simulink model "PositionComplementary2"  (Simulink 6.6)
settings: Solver=ode4  StartTime=0.0  StopTime=1800  FixedStep=SampleT  RelTol=1e-3
InitFcn:
  | clc
  | Taxi_Var_new
  | failures
  | insInit
  | piccolo_init
values from neighbouring files (symbols this model uses):
  A1 = 0    [Taxi_Var.m]    (also in Taxi_Var_new.m = 0.007)
  Apolar = 0.0899    [Taxi_Var.m]    (also in Taxi_Var_new.m = 0.057)
  CD0 = 0.0219    [Taxi_Var.m]    (also in Taxi_Var_new.m = 0.022)
  chord = S/span    (= 0.384036716878)    [Taxi_Var.m]    (also in Taxi_Var_new.m = 0.351341681574)
  CL0 = 0.1857    [Taxi_Var.m]    (also in Taxi_Var_new.m = 0.38)
  CLa = 4.6206    [Taxi_Var.m]    (also in Taxi_Var_new.m = 18.5)
  CLa_dot = 1.93    [Taxi_Var.m]    (also in Taxi_Var_new.m = 2.64)
  Clb = -0.0043    [Taxi_Var.m]    (also in Taxi_Var_new.m = -0.06)
  ClDa = 0.1695    [Taxi_Var.m]    (also in Taxi_Var_new.m)
  CLDe = 0.4032    [Taxi_Var.m]    (also in Taxi_Var_new.m = 0.24)
  CLDf = 0.047    [Taxi_Var.m]    (also in Taxi_Var_new.m = 0.4)
  ClDr = 0.0003    [Taxi_Var.m]    (also in Taxi_Var_new.m = 0.055)
  Clp = -0.4425    [Taxi_Var.m]    (also in Taxi_Var_new.m = -0.88)
  CLq = 8.7465    [Taxi_Var.m]    (also in Taxi_Var_new.m = 7.4)
  Clr = 0.0675    [Taxi_Var.m]    (also in Taxi_Var_new.m = 0.04)
  Cm0 = -0.0902    [Taxi_Var.m]    (also in Taxi_Var_new.m = 0.56)
  Cma = -1.3995    [Taxi_Var.m]    (also in Taxi_Var_new.m = -1.58)
  CmDe = -0.9493    [Taxi_Var.m]    (also in Taxi_Var_new.m = -41)
  CmDf = -.021    (= -0.021)    [Taxi_Var.m]    (also in Taxi_Var_new.m)
  Cmq = -10.8760    (= -10.876)    [Taxi_Var.m]    (also in Taxi_Var_new.m = -12)
  Cnb = 0.0281    [Taxi_Var.m]    (also in Taxi_Var_new.m = 0.73)
  CnDa = -0.0031    [Taxi_Var.m]    (also in Taxi_Var_new.m = -0.032)
  CnDr = -0.0882    [Taxi_Var.m]    (also in Taxi_Var_new.m = 0.19)
  Cnp = -0.0695    [Taxi_Var.m]    (also in Taxi_Var_new.m = -0.1)
  Cnr = -0.1045    [Taxi_Var.m]    (also in Taxi_Var_new.m = -0.23)
  CYb = -0.1999    [Taxi_Var.m]    (also in Taxi_Var_new.m = -0.98)
  CYDr = 0.0192    [Taxi_Var.m]    (also in Taxi_Var_new.m = 0.066)
  damax = 25*deg2rad    (= 0.436332312999)    [Taxi_Var.m]    (also in piccolo_init.m)
  damin = -25*deg2rad    (= -0.436332312999)    [Taxi_Var.m]    (also in piccolo_init.m)
  datrim = 0*deg2rad    (= 0)    [Taxi_Var.m]    (also in piccolo_init.m)
  demax = 15*deg2rad    (= 0.261799387799)    [Taxi_Var.m]    (also in piccolo_init.m)
  demin = -15*deg2rad    (= -0.261799387799)    [Taxi_Var.m]    (also in piccolo_init.m)
  detrim = -2.4137*deg2rad    (= -0.0421270121554)    [Taxi_Var.m]    (also in piccolo_init.m = -0.0523598775598)
  dfland = 30*deg2rad    (= 0.523598775598)    [Taxi_Var.m]    (also in piccolo_init.m)
  dfmax = 30*deg2rad    (= 0.523598775598)    [Taxi_Var.m]    (also in piccolo_init.m)
  dfmin = 0*deg2rad    (= 0)    [Taxi_Var.m]    (also in piccolo_init.m)
  drmax = 25*deg2rad    (= 0.436332312999)    [Taxi_Var.m]    (also in piccolo_init.m)
  drmin = -25*deg2rad    (= -0.436332312999)    [Taxi_Var.m]    (also in piccolo_init.m)
  drtrim = 0*deg2rad    (= 0)    [Taxi_Var.m]    (also in piccolo_init.m)
  dtmax = 1    [Taxi_Var.m]    (also in piccolo_init.m = 0.7)
  dtmin = 0    [Taxi_Var.m]    (also in piccolo_init.m = 0.25)
  dttrim = 0.0725    [Taxi_Var.m]    (also in piccolo_init.m = 0.35)
  Euler_0 = [0; 0; 45]'*pi/180    [Taxi_Var.m]    (also in Taxi_Var_new.m = [0 0 45]'*pi/180)
  IdxCmdOrbitRadius = 17    [piccolo_init.m]
  IdxCmdOrbitSense = 18    [piccolo_init.m]
  IdxCmdWp1Alt = 13    [piccolo_init.m]
  IdxCmdWp1Lat = 11    [piccolo_init.m]
  IdxCmdWp1Lon = 12    [piccolo_init.m]
  IdxCmdWp2Alt = 16    [piccolo_init.m]
  IdxCmdWp2Lat = 14    [piccolo_init.m]
  IdxCmdWp2Lon = 15    [piccolo_init.m]
  IdxEstimReserved1 = 4    [piccolo_init.m]
  IdxEstimWEast = 3    [piccolo_init.m]
  IdxEstimWNorth = 2    [piccolo_init.m]
  IdxGainsAltD = 10    [piccolo_init.m]
  IdxGainsAltI = 9    [piccolo_init.m]
  IdxGainsAltP = 8    [piccolo_init.m]
  IdxGainsPdynD = 4    [piccolo_init.m]
  IdxGainsPdynI = 3    [piccolo_init.m]
  IdxGainsPdynP = 2    [piccolo_init.m]
  IdxGainsPitchD = 7    [piccolo_init.m]
  IdxGainsPitchI = 6    [piccolo_init.m]
  IdxGainsPitchP = 5    [piccolo_init.m]
  IdxGainsRollD = 17    [piccolo_init.m]
  IdxGainsRollI = 16    [piccolo_init.m]
  IdxGainsRollP = 15    [piccolo_init.m]
  IdxGainsSlopeElevatorD = 25    [piccolo_init.m]
  IdxGainsSlopeElevatorP = 26    [piccolo_init.m]
  IdxGainsTrackConv = 24    [piccolo_init.m]
  IdxGainsTrackD = 23    [piccolo_init.m]
  IdxGainsTrackI = 22    [piccolo_init.m]
  IdxGainsTrackP = 21    [piccolo_init.m]
  IdxGainsTurnD = 14    [piccolo_init.m]
  IdxGainsTurnI = 13    [piccolo_init.m]
  IdxGainsTurnP = 12    [piccolo_init.m]
  IdxGainsYawD = 20    [piccolo_init.m]
  IdxGainsYawI = 19    [piccolo_init.m]
  IdxGainsYawP = 18    [piccolo_init.m]
  IdxLimitsAileronMax = 11    [piccolo_init.m]
  IdxLimitsAileronMin = 10    [piccolo_init.m]
  IdxLimitsBankMax = 9    [piccolo_init.m]
  IdxLimitsBankMin = 8    [piccolo_init.m]
  IdxLimitsElevatorMax = 13    [piccolo_init.m]
  IdxLimitsElevatorMin = 12    [piccolo_init.m]
  IdxLimitsFlapMax = 19    [piccolo_init.m]
  IdxLimitsFlapMin = 18    [piccolo_init.m]
  IdxLimitsPdynMax = 3    [piccolo_init.m]
  IdxLimitsPdynMin = 2    [piccolo_init.m]
  IdxLimitsRudderMax = 15    [piccolo_init.m]
  IdxLimitsRudderMin = 14    [piccolo_init.m]
  IdxLimitsThrottleMax = 17    [piccolo_init.m]
  IdxLimitsThrottleMin = 16    [piccolo_init.m]
  IdxSensorsAlt = 5    [piccolo_init.m]
  IdxSensorsLat = 3    [piccolo_init.m]
  IdxSensorsLon = 4    [piccolo_init.m]
  IdxSensorsVDown = 8    [piccolo_init.m]
  IdxSensorsVEast = 7    [piccolo_init.m]
  IdxSensorsVNorth = 6    [piccolo_init.m]
  IdxStatesGlobal = 2    [piccolo_init.m]
  IdxStatesManual = 16    [piccolo_init.m]
  IdxStatesMode = 15    [piccolo_init.m]
  ISA_g = 9.815    [Taxi_Var.m]    (also in Taxi_Var_new.m)
  ISA_hmax = 2000    [Taxi_Var.m]    (also in Taxi_Var_new.m)
  ISA_lapse = .0065    (= 0.0065)    [Taxi_Var.m]    (also in Taxi_Var_new.m)
  ISA_P0 = 101325    [Taxi_Var.m]    (also in Taxi_Var_new.m)
  ISA_R = 287    [Taxi_Var.m]    (also in Taxi_Var_new.m)
  ISA_rho0 = 1.225    [Taxi_Var.m]    (also in Taxi_Var_new.m)
  ISA_T0 = 289    [Taxi_Var.m]    (also in Taxi_Var_new.m)
  Ixx = 3.689084    [Taxi_Var.m]    (also in Taxi_Var_new.m = 3.8)
  Iyy = 7.43789    [Taxi_Var.m]    (also in Taxi_Var_new.m = 9.58)
  Izz = 10.22202    [Taxi_Var.m]    (also in Taxi_Var_new.m = 9.68)
  mass = 22.5    [Taxi_Var.m]    (also in Taxi_Var_new.m = 8.16466266)
  MinThK = 0.075    [Taxi_Var.m]    (also in Taxi_Var_new.m = 0.077)
  Pos_0 = [0; 0; 1000]'    [Taxi_Var.m]    (also in Taxi_Var_new.m = [0 0 500]')
  PQR_0 = [0; 0; 0]'    [Taxi_Var.m]    (also in Taxi_Var_new.m = [ 0 0 0]'*pi/180)
  SampleT = 0.005    [failures.m]
  span = 2.3368    [Taxi_Var.m]    (also in Taxi_Var_new.m = 2.795)
  TFact = 0.4    [Taxi_Var.m]    (also in Taxi_Var_new.m)
  ThK = 2.18    [Taxi_Var.m]    (also in Taxi_Var_new.m = 2.17)
  tsamp = APtsamp    (= 0.05)    [piccolo_init.m]
  ... (+1 more)
undefined symbols (not defined in the file or in its folder): clock, DiscIntNeverNeededParam, Earth, gaind, polesd, WGS84, zerosd
libraries: piccolo_library x60, simulink x49, aerolibconvert2 x16, dspsigops x5, aerolibasang x5, aerolibatmos2 x2, aerolibtransform2 x2, aerolibnav x2, aerolibutil x1, dspmtrx3 x1
(part 2 of 6)

== system PositionComplementary2/Subsystem3/Autopilot ==
  Sensors : Inport  PortDimensions=SizeSensors
  Estimates : Inport  Port=2  PortDimensions=SizeEstim
  Settings : Inport  Port=3  PortDimensions=SizeSet
  Commands : Inport  Port=4  PortDimensions=SizeCmd
  States : Inport  Port=5  PortDimensions=SizeStates
  Gains : Inport  Port=6  PortDimensions=SizeGains
  Limits : Inport  Port=7  PortDimensions=SizeLimits
  Autopilot Enable : EnablePort  StatesWhenEnabling=reset
  Air System Vector Inputs : piccolo_library/Flight Mechanics/Air System Vector Inputs  SystemSampleTime=-1  tsamp=APtsamp
  Altitude Control Vector Inputs : Subsystem  AncestorBlock=piccolo_library/Controllers/Longitudinal/Altitude Control Vector Inputs
  Demux{,1..6} (7 alike) : Demux  Outputs=7
  Flap Control Vector Inputs : Subsystem
  Gain : Gain  SaturateOnIntegerOverflow=on
  Gain1 : Gain  SaturateOnIntegerOverflow=on
  Guidance & Navigation Vector Input : Subsystem  AncestorBlock=piccolo_library/Controllers/Guidance/Guidance & Navigation Vector Input
  Mux : Mux  Inputs=12
  Mux1 : Mux  Inputs=5
  Mux2 : Mux  Inputs=7
  Pitch Control  Vector Inputs : Subsystem  AncestorBlock="piccolo_library/Controllers/Longitudinal/Pitch Control  Vector Inputs"
  Reserved Outputs : Constant  Value=0
  Roll Control Vector Inputs : Subsystem  AncestorBlock=piccolo_library/Controllers/Lateral/Roll Control Vector Inputs
  Yaw Control Vector Inputs : Subsystem  AncestorBlock=piccolo_library/Controllers/Lateral/Yaw Control Vector Inputs
  Actuators : Outport  OutDataType=fixdt(1,16,0)  OutScaling=[]
  Derived : Outport  Port=2  OutDataType=fixdt(1,16,0)  OutScaling=[]
  NPSTrim : Outport  Port=3  OutDataType=fixdt(1,16,0)  OutScaling=[]  InitialOutput=0
  wires:
  Mux/1 -> Gain/1, NPSTrim/1
  Mux1/1 -> Roll Control Vector Inputs/8(Derived), Altitude Control Vector Inputs/8(Derived), Pitch Control  Vector Inputs/8(Derived), Guidance & Navigation Vector Input/8(Derived), Yaw Control Vector Inputs/8(Derived), Air System Vector Inputs/8, Flap Control Vector Inputs/8(Derived), Gain1/1
  Roll Control Vector Inputs/1(Actuator) -> Mux/2
  Pitch Control  Vector Inputs/1(Actuator) -> Mux/4
  Altitude Control Vector Inputs/1(Actuator) -> Mux/8
  Sensors/1 -> Mux2/1
  Estimates/1 -> Mux2/2
  Settings/1 -> Mux2/3
  Commands/1 -> Mux2/4
  States/1 -> Mux2/5
  Gains/1 -> Mux2/6
  Limits/1 -> Mux2/7
  Demux/1 -> Altitude Control Vector Inputs/1(Sensors)
  Demux/2 -> Altitude Control Vector Inputs/2(Estimates)
  Demux/3 -> Altitude Control Vector Inputs/3(Settings)
  Demux/4 -> Altitude Control Vector Inputs/4(Commands)
  Demux/5 -> Altitude Control Vector Inputs/5(States)
  Demux/6 -> Altitude Control Vector Inputs/6(Gains)
  Demux/7 -> Altitude Control Vector Inputs/7(Limits)
  Demux1/1 -> Roll Control Vector Inputs/1(Sensors)
  Demux1/2 -> Roll Control Vector Inputs/2(Estimates)
  Demux1/3 -> Roll Control Vector Inputs/3(Settings)
  Demux1/4 -> Roll Control Vector Inputs/4(Commands)
  Demux1/5 -> Roll Control Vector Inputs/5(States)
  Demux1/6 -> Roll Control Vector Inputs/6(Gains)
  Demux1/7 -> Roll Control Vector Inputs/7(Limits)
  Demux2/1 -> Pitch Control  Vector Inputs/1(Sensors)
  Demux2/2 -> Pitch Control  Vector Inputs/2(Estimates)
  Demux2/3 -> Pitch Control  Vector Inputs/3(Settings)
  Demux2/4 -> Pitch Control  Vector Inputs/4(Commands)
  Demux2/5 -> Pitch Control  Vector Inputs/5(States)
  Demux2/6 -> Pitch Control  Vector Inputs/6(Gains)
  Demux2/7 -> Pitch Control  Vector Inputs/7(Limits)
  Demux3/1 -> Guidance & Navigation Vector Input/1(Sensors)
  Demux3/2 -> Guidance & Navigation Vector Input/2(Estimates)
  Demux3/3 -> Guidance & Navigation Vector Input/3(Settings)
  Demux3/4 -> Guidance & Navigation Vector Input/4(Commands)
  Demux3/5 -> Guidance & Navigation Vector Input/5(States)
  Demux3/6 -> Guidance & Navigation Vector Input/6(Gains)
  Demux3/7 -> Guidance & Navigation Vector Input/7(Limits)
  Demux4/1 -> Yaw Control Vector Inputs/1(Sensors)
  Demux4/2 -> Yaw Control Vector Inputs/2(Estimates)
  Demux4/3 -> Yaw Control Vector Inputs/3(Settings)
  Demux4/4 -> Yaw Control Vector Inputs/4(Commands)
  Demux4/5 -> Yaw Control Vector Inputs/5(States)
  Demux4/6 -> Yaw Control Vector Inputs/6(Gains)
  Demux4/7 -> Yaw Control Vector Inputs/7(Limits)
  Demux5/1 -> Air System Vector Inputs/1
  Demux5/2 -> Air System Vector Inputs/2
  Demux5/3 -> Air System Vector Inputs/3
  Demux5/4 -> Air System Vector Inputs/4
  Demux5/5 -> Air System Vector Inputs/5
  Demux5/6 -> Air System Vector Inputs/6
  Demux5/7 -> Air System Vector Inputs/7
  Mux2/1 -> Demux1/1, Demux/1, Demux2/1, Demux3/1, Demux4/1, Demux5/1, Demux6/1
  Reserved Outputs/1 -> Mux/11, Mux/9, Mux/7, Mux/1, Mux/3, Mux/5, Mux/12
  Yaw Control Vector Inputs/1(Actuator) -> Mux/6
  Flap Control Vector Inputs/1(Actuator) -> Mux/10
  Demux6/1 -> Flap Control Vector Inputs/1(Sensors)
  Demux6/2 -> Flap Control Vector Inputs/2(Estimates)
  Demux6/3 -> Flap Control Vector Inputs/3(Settings)
  Demux6/4 -> Flap Control Vector Inputs/4(Commands)
  Demux6/5 -> Flap Control Vector Inputs/5(States)
  Demux6/6 -> Flap Control Vector Inputs/6(Gains)
  Demux6/7 -> Flap Control Vector Inputs/7(Limits)
  Air System Vector Inputs/1 -> Mux1/1
  Roll Control Vector Inputs/2(Param) -> Mux1/2
  Pitch Control  Vector Inputs/2(Param) -> Mux1/3
  Guidance & Navigation Vector Input/1(Param) -> Mux1/4
  Altitude Control Vector Inputs/2(Param) -> Mux1/5
  Gain/1 -> Actuators/1
  Gain1/1 -> Derived/1

== system PositionComplementary2/Subsystem3/L1 Adaptive Controller LATERAL-DIRECTIONAL ==
  u_psi_c : Inport
  u_psi : Inport  Port=2
  Display : Display
  Mux2 : Mux  Inputs=2
  PF Yaw Channel L1 Augmentation : Subsystem  Orientation=left
  Scope1 : Scope  NumInputPorts=2
      settings: YMin=0.0999875~-4.5e-005  YMax=0.100045~1.25e-005  SaveName=ScopeData28
  Sum1 : Sum  Inputs=-+|
  Sum2 : Sum  Inputs=-+|
  u2 : Outport
  wires:
  u_psi/1 -> PF Yaw Channel L1 Augmentation/1(u_psi), Mux2/2, Sum2/1
  PF Yaw Channel L1 Augmentation/1(C_sighat_2) -> Sum1/1, Display/1  "L1 augmentation"
  u_psi_c/1 -> Sum1/2, Mux2/1, Sum2/2
  Sum1/1 -> u2/1, PF Yaw Channel L1 Augmentation/2(u2)
  Mux2/1 -> Scope1/1
  Sum2/1 -> Scope1/2

== system PositionComplementary2/Subsystem3/L1 Adaptive Controller LONGITUDINAL ==
  u_psi_c : Inport
  u_psi : Inport  Port=2
  Display : Display
  Mux2 : Mux  Inputs=2
  PF Yaw Channel L1 Augmentation : Subsystem  Orientation=left
  Scope1 : Scope  NumInputPorts=2
      settings: YMin=0.0999875~-4.5e-005  YMax=0.100045~1.25e-005  SaveName=ScopeData28
  Sum1 : Sum  Inputs=-+|
  Sum2 : Sum  Inputs=-+|
  u2 : Outport
  wires:
  Sum2/1 -> Scope1/2
  Mux2/1 -> Scope1/1
  Sum1/1 -> PF Yaw Channel L1 Augmentation/2(u2), u2/1
  u_psi_c/1 -> Sum2/2, Mux2/1, Sum1/2
  PF Yaw Channel L1 Augmentation/1(C_sighat_2) -> Display/1, Sum1/1  "L1 augmentation"
  u_psi/1 -> Sum2/1, Mux2/2, PF Yaw Channel L1 Augmentation/1(u_psi)

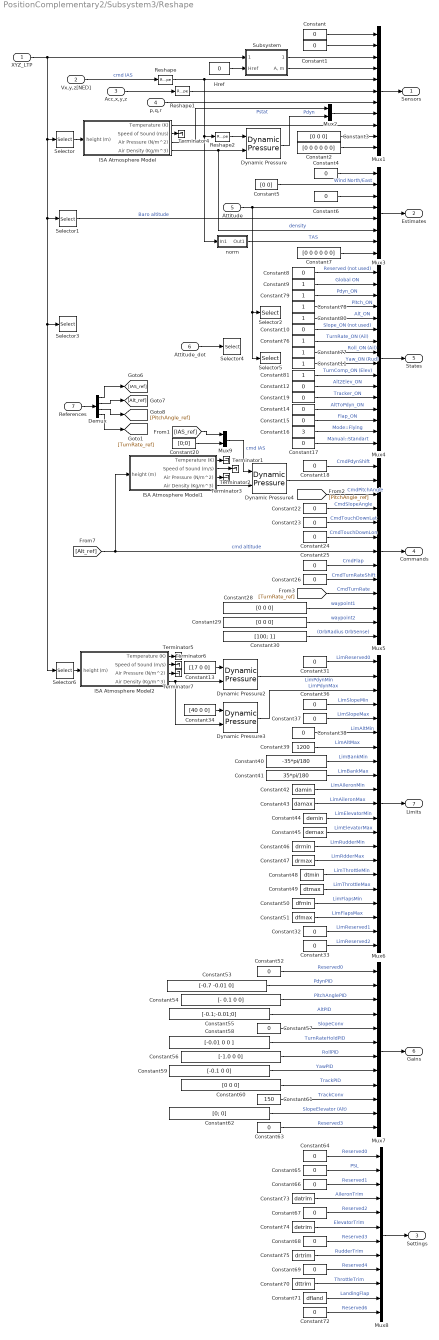
== system PositionComplementary2/Subsystem3/Reshape ==
  XYZ_LTP : Inport  OutDataType=fixdt(1,16,0)  OutScaling=[]
  Vx,y,z[NED] : Inport  Port=2  OutDataType=fixdt(1,16,0)  OutScaling=[]
  Acc,x,y,z : Inport  Port=3  OutDataType=fixdt(1,16,0)  OutScaling=[]
  p,q,r : Inport  Port=4  OutDataType=fixdt(1,16,0)  OutScaling=[]
  Attitude : Inport  Port=5  OutDataType=fixdt(1,16,0)  OutScaling=[]
  Attitude_dot : Inport  Port=6  OutDataType=fixdt(1,16,0)  OutScaling=[]
  References : Inport  Port=7  OutDataType=fixdt(1,16,0)  OutScaling=[]
  Constant{,1,4,6,8,10,12,14..15,17..19,22..26,31..33,36..38,52,57,63..69,72} (33 alike) : Constant  Value=0
  Constant{9,11,76..81} (8 alike) : Constant
  Constant13 : Constant  Value=[17 0 0]
  Constant16 : Constant  Value=3
  Constant2 : Constant  Value=[0 0 0 0 0 0]
  Constant20 : Constant  Value=[0;0]
  Constant{3,28..29,60} (4 alike) : Constant  Value=[0 0 0]
  Constant30 : Constant  Value=[100; 1]
  Constant34 : Constant  Value=[40 0 0]
  Constant39 : Constant  Value=1200
  Constant40 : Constant  Value=-35*pi/180
  Constant41 : Constant  Value=35*pi/180
  Constant42 : Constant  Value=damin
  Constant43 : Constant  Value=damax
  Constant44 : Constant  Value=demin
  Constant45 : Constant  Value=demax
  Constant46 : Constant  Value=drmin
  Constant47 : Constant  Value=drmax
  Constant48 : Constant  Value=dtmin
  Constant49 : Constant  Value=dtmax
  Constant5 : Constant  Value=[0 0]
  Constant50 : Constant  Value=dfmin
  Constant51 : Constant  Value=dfmax
  Constant53 : Constant  Value=[-0.7 -0.01 0]
  Constant54 : Constant  Value=[- 0.1 0 0]
  Constant55 : Constant  Value=[-0.1;-0.01;0]
  Constant56 : Constant  Value=[-1.0 0 0]
  Constant58 : Constant  Value=[-0.01 0 0 ]
  Constant59 : Constant  Value=[-0.1 0 0]
  Constant61 : Constant  Value=150
  Constant62 : Constant  Value=[0; 0]
  Constant7 : Constant  Value=[0 0 0 0 0 0]
  Constant70 : Constant  Value=dttrim
  Constant71 : Constant  Value=dfland
  Constant73 : Constant  Value=datrim
  Constant74 : Constant  Value=detrim
  Constant75 : Constant  Value=drtrim
  Demux : Demux
  Dynamic Pressure{,2..4} (4 alike) : aerolibasang/Dynamic Pressure  SystemSampleTime=-1
  Href : Constant  Value=0
  ISA Atmosphere Model : Subsystem  mask(International Standart Atmosphere){L=ISA_lapse, h_lim=ISA_hmax, R=ISA_R, g=ISA_g, rh0=ISA_rho0, P0=ISA_P0, T0=ISA_T0}
      mask prompts: L "Lapse rate"; h_lim "Upper altitude limit, (m)"; R "Universal gas constant R"; g "Garvity constant, (m/c^2)"; rh0 "Sea level density, (kg/m^3)"; P0 "Sea level pressure, (N/m^2)"; T0 "Sea level temperature, (K)"
  ISA Atmosphere Model1 : Subsystem  mask(International Standart Atmosphere){L=ISA_lapse, h_lim=ISA_hmax, R=ISA_R, g=ISA_g, rh0=ISA_rho0, P0=ISA_P0, T0=ISA_T0}
      mask prompts: L "Lapse rate"; h_lim "Upper altitude limit, (m)"; R "Universal gas constant R"; g "Garvity constant, (m/c^2)"; rh0 "Sea level density, (kg/m^3)"; P0 "Sea level pressure, (N/m^2)"; T0 "Sea level temperature, (K)"
  ISA Atmosphere Model2 : Subsystem  mask(International Standart Atmosphere){L=ISA_lapse, h_lim=ISA_hmax, R=ISA_R, g=ISA_g, rh0=ISA_rho0, P0=ISA_P0, T0=ISA_T0}
      mask prompts: L "Lapse rate"; h_lim "Upper altitude limit, (m)"; R "Universal gas constant R"; g "Garvity constant, (m/c^2)"; rh0 "Sea level density, (kg/m^3)"; P0 "Sea level pressure, (N/m^2)"; T0 "Sea level temperature, (K)"
  Mux1 : Mux  Inputs=11
  Mux2 : Mux  Inputs=2
  Mux3 : Mux  Inputs=8
  Mux4 : Mux  Inputs=16
  Mux5 : Mux  Inputs=13
  Mux6 : Mux  Inputs=21
  Mux7 : Mux  Inputs=12
  Mux8 : Mux  Inputs=12
  Mux9 : Mux  Inputs=2
  Reshape : Reshape
  Reshape1 : Reshape
  Reshape2 : Reshape
  Selector{,1,3..4,6} (5 alike) : Selector  IndexOptions=Index vector (dialog)  Indices=3  OutputSizes=[(-2)]  InputPortWidth=3
  Selector2 : Selector  IndexOptions=Index vector (dialog)  Indices=2  OutputSizes=[(-2)]  InputPortWidth=3
  Selector5 : Selector  IndexOptions=Index vector (dialog)  Indices=[1 3]  OutputSizes=[(-2)]  InputPortWidth=3
  Subsystem : Subsystem
  Terminator{1..7} (7 alike) : Terminator
  norm : Subsystem
  Sensors : Outport  OutDataType=fixdt(1,16,0)  OutScaling=[]
  Estimates : Outport  Port=2  OutDataType=fixdt(1,16,0)  OutScaling=[]
  Settings : Outport  Port=3  OutDataType=fixdt(1,16,0)  OutScaling=[]
  Commands : Outport  Port=4  OutDataType=fixdt(1,16,0)  OutScaling=[]
  States : Outport  Port=5  OutDataType=fixdt(1,16,0)  OutScaling=[]
  Gains : Outport  Port=6  OutDataType=fixdt(1,16,0)  OutScaling=[]
  Limits : Outport  Port=7  OutDataType=fixdt(1,16,0)  OutScaling=[]
  wires:
  Constant/1 -> Mux1/1
  Constant1/1 -> Mux1/2
  Subsystem/1("LL, deg") -> Mux1/3
  Subsystem/2("A, m") -> Mux1/4
  XYZ_LTP/1 -> Subsystem/1("XYZ, ltp"), Selector/1, Selector1/1, Selector3/1, Selector6/1
  Vx,y,z[NED]/1 -> Reshape/1  "cmd IAS"
  Mux1/1 -> Sensors/1
  Acc,x,y,z/1 -> Reshape1/1
  p,q,r/1 -> Mux1/7
  Constant3/1 -> Mux1/10
  Constant2/1 -> Mux1/11
  ISA Atmosphere Model/4(Air Density (Kg/m^3)) -> Dynamic Pressure/2, Mux3/6  "density"
  ISA Atmosphere Model/1(Temperature (K)) -> Mux1/9
  Mux2/1 -> Mux1/8
  ISA Atmosphere Model/3("Air Pressure (N/m^2) ") -> Mux2/1  "Pstat"
  ISA Atmosphere Model/2("Speed of Sound (m/s) ") -> Terminator4/1
  Dynamic Pressure/1 -> Mux2/2  "Pdyn"
  Selector/1 -> ISA Atmosphere Model/1(height (m))
  Reshape/1 -> Mux1/5, Reshape2/1, norm/1(In1)
  Reshape1/1 -> Mux1/6
  Reshape2/1 -> Dynamic Pressure/1
  Href/1 -> Subsystem/2(Href)
  Mux3/1 -> Estimates/1
  Constant4/1 -> Mux3/1
  Constant5/1 -> Mux3/2  "Wind North/East"
  Constant6/1 -> Mux3/3
  Attitude/1 -> Selector2/1, Selector5/1, Mux3/4
  Selector1/1 -> Mux3/5  "Baro altitude"
  norm/1(Out1) -> Mux3/7  "TAS"
  Constant7/1 -> Mux3/8
  Mux4/1 -> States/1
  Constant8/1 -> Mux4/1  "Reserved (not used)"
  Constant9/1 -> Mux4/2  "Global ON"
  Constant10/1 -> Mux4/6  "Slope_ON (not used)"
  Attitude_dot/1 -> Selector4/1
  Constant11/1 -> Mux4/9  "Yaw_ON (Rud)"
  Mux5/1 -> Commands/1
  Constant18/1 -> Mux5/1  "CmdPdynShift"
  ISA Atmosphere Model1/1(Temperature (K)) -> Terminator1/1
  ISA Atmosphere Model1/2("Speed of Sound (m/s) ") -> Terminator2/1
  ISA Atmosphere Model1/3("Air Pressure (N/m^2) ") -> Terminator3/1
  ISA Atmosphere Model1/4(Air Density (Kg/m^3)) -> Dynamic Pressure4/2
  Dynamic Pressure4/1 -> Mux5/2
  Mux9/1 -> Dynamic Pressure4/1  "cmd IAS"
  [Alt_ref] -> ISA Atmosphere Model1/1(height (m)), Mux5/7  "cmd altitude"
  [PitchAngle_ref] -> Mux5/3  "CmdPitchAngle"
  Constant22/1 -> Mux5/4  "CmdSlopeAngle"
  Constant24/1 -> Mux5/6  "CmdTouchDownLon"
  Constant23/1 -> Mux5/5  "CmdTouchDownLat"
  Constant25/1 -> Mux5/8  "CmdFlap"
  Constant26/1 -> Mux5/9  "CmdTurnRateShift"
  [TurnRate_ref] -> Mux5/10  "CmdTurnRate"
  Constant28/1 -> Mux5/11  "waypoint1"
  Constant29/1 -> Mux5/12  "waypoint2"
  Constant30/1 -> Mux5/13  "(OrbRadius OrbSense)"
  Mux6/1 -> Limits/1
  Constant31/1 -> Mux6/1  "LimReserved0"
  Constant33/1 -> Mux6/21  "LimReserved2"
  Constant32/1 -> Mux6/20  "LimReserved1"
  ISA Atmosphere Model2/1(Temperature (K)) -> Terminator5/1
  ISA Atmosphere Model2/2("Speed of Sound (m/s) ") -> Terminator6/1
  ISA Atmosphere Model2/3("Air Pressure (N/m^2) ") -> Terminator7/1
  ISA Atmosphere Model2/4(Air Density (Kg/m^3)) -> Dynamic Pressure2/2, Dynamic Pressure3/2
  Constant13/1 -> Dynamic Pressure2/1
  Constant34/1 -> Dynamic Pressure3/1
  Selector6/1 -> ISA Atmosphere Model2/1(height (m))
  Dynamic Pressure2/1 -> Mux6/2  "LimPdynMin"
  Dynamic Pressure3/1 -> Mux6/3  "LimPdynMax"
  Constant36/1 -> Mux6/4  "LimSlopeMin"
  Constant37/1 -> Mux6/5  "LimSlopeMax"
  Constant38/1 -> Mux6/6  "LimAltMin"
  Constant39/1 -> Mux6/7  "LimAltMax"
  Constant40/1 -> Mux6/8  "LimBankMin"
  Constant41/1 -> Mux6/9  "LimBankMax"
  Constant42/1 -> Mux6/10  "LimAileronMin"
  Constant43/1 -> Mux6/11  "LimAileronMax"
  Constant44/1 -> Mux6/12  "LimElevatorMin"
  Constant45/1 -> Mux6/13  "LimElevatorMax"
  Constant46/1 -> Mux6/14  "LimRudderMin"
  Constant47/1 -> Mux6/15  "LimRdderMax"
  Constant48/1 -> Mux6/16  "LimThrottleMin"
  Constant49/1 -> Mux6/17  "LimThrottleMax"
  Constant50/1 -> Mux6/18  "LimFlapsMin"
  Constant51/1 -> Mux6/19  "LimFlapsMax"
  Mux7/1 -> Gains/1
  Constant52/1 -> Mux7/1  "Reserved0"
  Constant53/1 -> Mux7/2  "PdynPID"
  Constant54/1 -> Mux7/3  "PitchAnglePID"
  Constant55/1 -> Mux7/4  "AltPID"
  Constant58/1 -> Mux7/6  "TurnRateHoldPID"
  Constant57/1 -> Mux7/5  "SlopeConv"
  Constant56/1 -> Mux7/7  "RollPID"
  Constant59/1 -> Mux7/8  "YawPID"
  Constant60/1 -> Mux7/9  "TrackPID"
  Constant61/1 -> Mux7/10  "TrackConv"
  Constant62/1 -> Mux7/11  "SlopeElevator (Alt)"
  Constant63/1 -> Mux7/12  "Reserved3"
  Mux8/1 -> Settings/1
  Constant64/1 -> Mux8/1  "Reserved0"
  Constant65/1 -> Mux8/2  "PSL"
  Constant66/1 -> Mux8/3  "Reserved1"
  Constant67/1 -> Mux8/5  "Reserved2"
  Constant68/1 -> Mux8/7  "Reserved3"
  Constant69/1 -> Mux8/9  "Reserved4"
  Constant70/1 -> Mux8/10  "ThrottleTrim"
  Constant71/1 -> Mux8/11  "LandingFlap"
  Constant72/1 -> Mux8/12  "Reserved6"
  Constant73/1 -> Mux8/4  "AileronTrim"
  Constant74/1 -> Mux8/6  "ElevatorTrim"
  Constant75/1 -> Mux8/8  "RudderTrim"
  Constant76/1 -> Mux4/7  "TurnRate_ON (Ail)"
  Constant77/1 -> Mux4/8  "Roll_ON (Ail)"
  Constant78/1 -> Mux4/4  "Pitch_ON"
  Constant79/1 -> Mux4/3  "Pdyn_ON"
  Constant80/1 -> Mux4/5  "Alt_ON"
  Constant81/1 -> Mux4/10  "TurnComp_ON (Elev)"
  Constant12/1 -> Mux4/11  "Alt2Elev_ON"
  Constant19/1 -> Mux4/12  "Tracker_ON"
  Constant14/1 -> Mux4/13  "AltToPdyn_ON"
  Constant15/1 -> Mux4/14  "Flap_ON"
  Constant16/1 -> Mux4/15  "Mode::Flying"
  Constant17/1 -> Mux4/16  "Manual::Standart"
  References/1 -> Demux/1
  Demux/1 -> [IAS_ref]
  Demux/2 -> [Alt_ref]
  Demux/3 -> [PitchAngle_ref]
  Demux/4 -> [TurnRate_ref]
  Constant20/1 -> Mux9/2
  [IAS_ref] -> Mux9/1

== system PositionComplementary2/Attitude Complementary Filter/Subsystem/Get Roll, Pitch ==
  Ab : Inport
  Demux : Demux  Outputs=3
  Gain : Gain  Gain=-1
  Gain1 : Gain  Gain=-1
  Mux : Mux  Inputs=2
  Trigonometric Function1 : Trigonometry  Operator=atan2  SampleTime=T
  Trigonometric Function2 : Trigonometry  Operator=atan2  SampleTime=T
  "Phi, The" : Outport
  wires:
  Ab/1 -> Demux/1
  Mux/1 -> "Phi, The"/1
  Demux/3 -> Gain/1
  Gain/1 -> Trigonometric Function1/2, Trigonometric Function2/2
  Demux/2 -> Trigonometric Function1/1
  Trigonometric Function1/1 -> Gain1/1
  Gain1/1 -> Mux/1
  Trigonometric Function2/1 -> Mux/2
  Demux/1 -> Trigonometric Function2/1

== system PositionComplementary2/Attitude Complementary Filter/Subsystem/get Centripetal ==
  pqr : Inport  Orientation=left
  Vb : Inport  Orientation=left  Port=2
  3vector LPF : Subsystem  Orientation=left  mask{flpf=100}
      mask prompts: flpf "LowPass Freq"
      mask Display: droots([],-flpf,flpf)
  3x3 Cross Product : aerolibutil/3x3 Cross Product  Orientation=left  SystemSampleTime=-1
  Integer Delay : simulink/Discrete/Integer Delay  Orientation=left  vinit=0.0  samptime=-1  NumDelays=1
  Saturation : Saturate  Orientation=left  UpperLimit=20  LowerLimit=-20
  w x Vb : Outport  Orientation=left
  wires:
  Integer Delay/1 -> 3x3 Cross Product/2
  pqr/1 -> 3vector LPF/1(In1)
  Vb/1 -> Integer Delay/1
  3x3 Cross Product/1 -> Saturation/1  "w x Vb"
  3vector LPF/1(Out1) -> 3x3 Cross Product/1
  Saturation/1 -> w x Vb/1

== system PositionComplementary2/Get GPS in LTP/Geod2LTP2/ECEF2LTP (UEN) ==
  ECEF coordinates : Inport
  "Long, Lat" : Inport  Port=2
  Deg2R : Gain  Gain=pi/180  SaturateOnIntegerOverflow=on
  Demux3 : Demux  Outputs=2
  From Body to Universal1 : Subsystem
  Product1 : Product  Multiplication=Matrix(*)  SaturateOnIntegerOverflow=on  InputSameDT=on
  Out : Outport
  wires:
  "Long, Lat"/1 -> Deg2R/1
  Product1/1 -> Out/1
  Demux3/2 -> From Body to Universal1/2(lat)
  Demux3/1 -> From Body to Universal1/1(long)
  Deg2R/1 -> Demux3/1
  ECEF coordinates/1 -> Product1/2
  From Body to Universal1/1(DCM) -> Product1/1

== system PositionComplementary2/Get GPS in LTP/Geod2LTP2/Geod2ECEF ==
  "height, m" : Inport
  "lat, deg" : Inport  Port=2
  lon,deg : Inport  Port=3
  (Rh+h)cos(phi)*cos(lamb)=Xe : Product  Inputs=3  SaturateOnIntegerOverflow=on  InputSameDT=on
  (Rh+h)cos(phi)*sin(lamb)=Ye : Product  Inputs=3  SaturateOnIntegerOverflow=on  InputSameDT=on
  Deg2R : Gain  Gain=pi/180  SaturateOnIntegerOverflow=on
  "Deg2R " : Gain  Gain=pi/180  SaturateOnIntegerOverflow=on
  Product1 : Product  SaturateOnIntegerOverflow=on  InputSameDT=on
  Re=equatorial radius : Constant  Value=Re
  Rh : Product  Inputs=*/  SaturateOnIntegerOverflow=on  InputSameDT=on
  Rh(1-e^2) : Product  SaturateOnIntegerOverflow=on  InputSameDT=on
  Sum1 : Sum  Inputs=+-|  SaturateOnIntegerOverflow=on  InputSameDT=on
  Sum2 : Sum  SaturateOnIntegerOverflow=on  InputSameDT=on
      settings: AttributesFormatString=Rh+h
  Sum3 : Sum  Inputs=|+-  SaturateOnIntegerOverflow=on  InputSameDT=on
  Sum4 : Sum  SaturateOnIntegerOverflow=on  InputSameDT=on
      settings: AttributesFormatString=(1-e^2)Rh+h
  Ze : Product  SaturateOnIntegerOverflow=on  InputSameDT=on
  const : Constant
  const1 : Constant
  cos(lamb) : Trigonometry  Operator=cos
  cos(phi) : Trigonometry  Operator=cos
  eccentricity^2 : Subsystem
  f : Fcn  Expr=sqrt(u(1))
  sin(lamb) : Trigonometry
  sin(phi) : Trigonometry
  sin(phi)^2 : Product  SaturateOnIntegerOverflow=on  InputSameDT=on
  "Xe, m " : Outport
  "Ye, m " : Outport  Port=2
  "Ze, m " : Outport  Port=3
  wires:
  "lat, deg"/1 -> Deg2R/1
  sin(phi)/1 -> sin(phi)^2/1, sin(phi)^2/2, Ze/1
  f/1 -> Rh/2
  Re=equatorial radius/1 -> Rh/1
  Rh/1 -> Sum2/2, Rh(1-e^2)/2
  Product1/1 -> Sum1/2
  Sum1/1 -> f/1
  const/1 -> Sum1/1
  "height, m"/1 -> Sum4/2, Sum2/1
  eccentricity^2/1(e^2) -> Product1/1, Sum3/2
  sin(phi)^2/1 -> Product1/2
  const1/1 -> Sum3/1
  Sum3/1 -> Rh(1-e^2)/1  "1-e^2"
  Rh(1-e^2)/1 -> Sum4/1
  Sum4/1 -> Ze/2
  lon,deg/1 -> "Deg2R "/1
  cos(phi)/1 -> (Rh+h)cos(phi)*cos(lamb)=Xe/2, (Rh+h)cos(phi)*sin(lamb)=Ye/2
  cos(lamb)/1 -> (Rh+h)cos(phi)*cos(lamb)=Xe/3
  sin(lamb)/1 -> (Rh+h)cos(phi)*sin(lamb)=Ye/3
  Ze/1 -> "Ze, m "/1
  Deg2R/1 -> cos(phi)/1, sin(phi)/1
  "Deg2R "/1 -> cos(lamb)/1, sin(lamb)/1
  Sum2/1 -> (Rh+h)cos(phi)*sin(lamb)=Ye/1, (Rh+h)cos(phi)*cos(lamb)=Xe/1
  (Rh+h)cos(phi)*cos(lamb)=Xe/1 -> "Xe, m "/1
  (Rh+h)cos(phi)*sin(lamb)=Ye/1 -> "Ye, m "/1

== system PositionComplementary2/Get GPS in LTP/Geod2LTP2/Geod2ECEF1 ==
  "height, m" : Inport
  "lat, deg" : Inport  Port=2
  lon,deg : Inport  Port=3
  (Rh+h)cos(phi)*cos(lamb)=Xe : Product  Inputs=3  SaturateOnIntegerOverflow=on  InputSameDT=on
  (Rh+h)cos(phi)*sin(lamb)=Ye : Product  Inputs=3  SaturateOnIntegerOverflow=on  InputSameDT=on
  Deg2R : Gain  Gain=pi/180  SaturateOnIntegerOverflow=on
  "Deg2R " : Gain  Gain=pi/180  SaturateOnIntegerOverflow=on
  Product1 : Product  SaturateOnIntegerOverflow=on  InputSameDT=on
  Re=equatorial radius : Constant  Value=Re
  Rh : Product  Inputs=*/  SaturateOnIntegerOverflow=on  InputSameDT=on
  Rh(1-e^2) : Product  SaturateOnIntegerOverflow=on  InputSameDT=on
  Sum1 : Sum  Inputs=+-|  SaturateOnIntegerOverflow=on  InputSameDT=on
  Sum2 : Sum  SaturateOnIntegerOverflow=on  InputSameDT=on
      settings: AttributesFormatString=Rh+h
  Sum3 : Sum  Inputs=|+-  SaturateOnIntegerOverflow=on  InputSameDT=on
  Sum4 : Sum  SaturateOnIntegerOverflow=on  InputSameDT=on
      settings: AttributesFormatString=(1-e^2)Rh+h
  Ze : Product  SaturateOnIntegerOverflow=on  InputSameDT=on
  const : Constant
  const1 : Constant
  cos(lamb) : Trigonometry  Operator=cos
  cos(phi) : Trigonometry  Operator=cos
  eccentricity^2 : Subsystem
  f : Fcn  Expr=sqrt(u(1))
  sin(lamb) : Trigonometry
  sin(phi) : Trigonometry
  sin(phi)^2 : Product  SaturateOnIntegerOverflow=on  InputSameDT=on
  "Xe, m " : Outport
  "Ye, m " : Outport  Port=2
  "Ze, m " : Outport  Port=3
  wires:
  (Rh+h)cos(phi)*sin(lamb)=Ye/1 -> "Ye, m "/1
  (Rh+h)cos(phi)*cos(lamb)=Xe/1 -> "Xe, m "/1
  Sum2/1 -> (Rh+h)cos(phi)*cos(lamb)=Xe/1, (Rh+h)cos(phi)*sin(lamb)=Ye/1
  "Deg2R "/1 -> sin(lamb)/1, cos(lamb)/1
  Deg2R/1 -> sin(phi)/1, cos(phi)/1
  Ze/1 -> "Ze, m "/1
  sin(lamb)/1 -> (Rh+h)cos(phi)*sin(lamb)=Ye/3
  cos(lamb)/1 -> (Rh+h)cos(phi)*cos(lamb)=Xe/3
  cos(phi)/1 -> (Rh+h)cos(phi)*sin(lamb)=Ye/2, (Rh+h)cos(phi)*cos(lamb)=Xe/2
  lon,deg/1 -> "Deg2R "/1
  Sum4/1 -> Ze/2
  Rh(1-e^2)/1 -> Sum4/1
  Sum3/1 -> Rh(1-e^2)/1  "1-e^2"
  const1/1 -> Sum3/1
  sin(phi)^2/1 -> Product1/2
  eccentricity^2/1(e^2) -> Sum3/2, Product1/1
  "height, m"/1 -> Sum2/1, Sum4/2
  const/1 -> Sum1/1
  Sum1/1 -> f/1
  Product1/1 -> Sum1/2
  Rh/1 -> Rh(1-e^2)/2, Sum2/2
  Re=equatorial radius/1 -> Rh/1
  f/1 -> Rh/2
  sin(phi)/1 -> Ze/1, sin(phi)^2/2, sin(phi)^2/1
  "lat, deg"/1 -> Deg2R/1

== system PositionComplementary2/Plant Model/Plant/6-DOF EOM ==
  "[F,M]" : Inport
  Vb Corr : Inport  Orientation=left  Port=2
  Angular Rates : Integrator  InitialCondition=PQR_0'  LimitOutput=on  UpperSaturationLimit=10  LowerSaturationLimit=-10
  Demux1 : Demux  Outputs=[3 3]
  Euler Angles : Integrator  InitialCondition=Euler_0'
  Get Euler Dot : Subsystem
      mask Display:
      | port_label('input', 1, 'p, q, r')
      | port_label('input', 2, 'Euler')
      | port_label('output', 1, 'Euler_dot')
  Mux : Mux  Orientation=left  Inputs=[3;3]
  NED2NEU : Gain  Gain=[1 0 0;0 1 0;0 0 -1]  Multiplication=Matrix(K*u)  SaturateOnIntegerOverflow=on
  Position : Integrator  InitialCondition=Pos_0'
  RB2L * Vb : Product  Multiplication=Matrix(*)  SaturateOnIntegerOverflow=on  InputSameDT=on
  RB2LTP : Subsystem
  Velocities Body : Integrator  InitialCondition=Vb_0'  LimitOutput=on  UpperSaturationLimit=200  LowerSaturationLimit=-200
  "[V1,2,3,W1,2,3]" : Subsystem
  X,Y,Z (LTP) : Outport
  "Vx, Vy, Vz" : Outport  Port=2
  Euler : Outport  Port=3
  "p, q, r" : Outport  Orientation=left  Port=4
  Euler_dot : Outport  Port=5
  Vb : Outport  Port=6
  Ab : Outport  Port=7
  Ab meas : Outport  Port=8
  wires:
  "[V1,2,3,W1,2,3]"/1("Acc_meas ") -> Ab meas/1
  Euler Angles/1 -> "[V1,2,3,W1,2,3]"/2(Euler), Get Euler Dot/2(Euler), Euler/1, RB2LTP/1(Euler)
  Demux1/1 -> Ab/1, Velocities Body/1
  "[V1,2,3,W1,2,3]"/2(V*dot) -> Demux1/1
  Demux1/2 -> Angular Rates/1
  "[F,M]"/1 -> "[V1,2,3,W1,2,3]"/1("[F ; M]")
  RB2LTP/1(Rot) -> RB2L * Vb/1
  Velocities Body/1 -> Vb/1, RB2L * Vb/2
  Mux/1 -> "[V1,2,3,W1,2,3]"/3(V*)
  Position/1 -> X,Y,Z (LTP)/1
  Angular Rates/1 -> Get Euler Dot/1(p,q,r), Mux/2, "p, q, r"/1
  RB2L * Vb/1 -> NED2NEU/1, "Vx, Vy, Vz"/1  "NED"
  NED2NEU/1 -> Position/1
  Get Euler Dot/1(Euler_dot) -> Euler Angles/1, Euler_dot/1
  Vb Corr/1 -> Mux/1

== system PositionComplementary2/Plant Model/Plant/Engine Model ==
  dt : Inport
  Vmag : Inport  Port=2
  Constant4 : Constant  Value=0
  Get To1 : Subsystem
  Mux : Mux  Inputs=2
  Mux1 : Mux  Inputs=3
  Thrust Available (lbs) : Fcn  Expr=u(1) - 0.047*sqrt(u(1))*u(2)
  kg2N : Gain  Gain=ISA_g  SaturateOnIntegerOverflow=on
  lbs2kg : Gain  Gain=0.45359237  SaturateOnIntegerOverflow=on
  RPM : Outport
  Thrust : Outport  Port=2
  wires:
  Get To1/1(RPM) -> RPM/1
  dt/1 -> Get To1/1(dt)
  Get To1/2(To) -> Mux/1
  Mux/1 -> Thrust Available (lbs)/1
  Thrust Available (lbs)/1 -> lbs2kg/1
  Vmag/1 -> Mux/2
  Mux1/1 -> Thrust/1
  lbs2kg/1 -> kg2N/1
  Constant4/1 -> Mux1/2, Mux1/3
  kg2N/1 -> Mux1/1

== system PositionComplementary2/Plant Model/Plant/Forces and Moments ==
  Wind e : Inport
  Rho : Inport  Port=2
  "de, deg" : Inport  Port=3
  da,deg : Inport  Port=4
  "dr, deg" : Inport  Port=5
  "df, deg" : Inport  Port=6
  "Vx, Vy, Vz " : Inport  Port=7
  Euler : Inport  Port=8  PortDimensions=3
  p,q,r : Inport  Port=9
  Alpha/Beta : Subsystem
  Body Frame F & M : Subsystem
  Get Grav Force in Body : Subsystem
  Gravitational Force : Constant  Value=[0 0 mass*ISA_g]  VectorParams1D=off
  Mux : Mux  Inputs=2
  Mux1 : Mux  Inputs=2
  NED(u)2b : Subsystem
  Scope : Scope
      settings: SaveName=ScopeData5
  Selector : Selector  IndexOptions=Index vector (dialog)  Indices=3  OutputSizes=1  InputPortWidth=3
  Selector1 : Selector  Orientation=up  IndexOptions=Index vector (dialog)  Indices=3  OutputSizes=1  InputPortWidth=3
  Sum : Sum  Inputs=|++  SaturateOnIntegerOverflow=on
  Vair : Sum  Inputs=+-  SaturateOnIntegerOverflow=on  InputSameDT=on
  Airspeed : Outport
  Forces : Outport  Port=2
  Moments : Outport  Port=3
  Vb Corr : Outport  Port=4
  "aoa/betta, deg" : Outport  Port=5
  q : Outport  Port=6
  wires:
  Get Grav Force in Body/1(Grav Force (Body)) -> Sum/2
  Selector1/1 -> Mux1/2
  Mux1/1 -> Scope/1
  Selector/1 -> Mux1/1
  Mux/1 -> "aoa/betta, deg"/1
  Alpha/Beta/5(q) -> q/1
  "Vx, Vy, Vz "/1 -> Vair/1
  Vair/1 -> NED(u)2b/1(V w)
  Euler/1 -> NED(u)2b/2(Euler), Get Grav Force in Body/1(Euler)
  Rho/1 -> Alpha/Beta/2(Rho)
  NED(u)2b/1(Vb Corr) -> Alpha/Beta/1("Vx, Vy, Vz (Body)"), Vb Corr/1
  Body Frame F & M/2(M_b) -> Moments/1
  Gravitational Force/1 -> Get Grav Force in Body/2(Grav Force)
  Body Frame F & M/1(F_b) -> Selector/1, Sum/1
  Sum/1 -> Selector1/1, Forces/1
  Alpha/Beta/3(qS) -> Body Frame F & M/3(qs)
  Alpha/Beta/4(Speed) -> Body Frame F & M/4(Airspeed), Airspeed/1
  "df, deg"/1 -> Body Frame F & M/8("df, deg")
  p,q,r/1 -> Body Frame F & M/9(p,q,r)
  Alpha/Beta/2("beta, deg") -> Mux/2, Body Frame F & M/2("Beta, deg")
  "dr, deg"/1 -> Body Frame F & M/7("dr, deg")
  da,deg/1 -> Body Frame F & M/6("da, deg")
  Alpha/Beta/1("alpha, deg") -> Mux/1, Body Frame F & M/1("Alpha, deg")
  "de, deg"/1 -> Body Frame F & M/5("de, deg")
  Wind e/1 -> Vair/2

== system PositionComplementary2/Plant Model/Plant/Get GPS ==
  XYZ (NEU) : Inport
  Angle Conversion : aerolibconvert2/Angle Conversion  SystemSampleTime=-1  IU=deg  OU=rad
  Demux : Demux  Outputs=6
  Demux2 : Demux  Outputs=2
  Flat Earth to LLA : aerolibtransform2/Flat Earth to LLA  SystemSampleTime=-1  units=Metric (MKS)  ptype=Earth (WGS84)  F=1/298.257223563  R=6378137  LL0=[37.0004768371582, -122.061897277832]  psi=0
  MATLAB Fcn : MATLABFcn  MATLABFcn=u(1)*clock  OutputSignalType=real
  NEU2NED : Gain  Gain=[1 0 0;0 1 0;0 0 -1]  Multiplication=Matrix(K*u)  SaturateOnIntegerOverflow=on
  Rounding Function : Rounding
  Zero level trust : Constant  Value=0
  Zero level trust1 : Constant
  Zero level trust2 : Constant  Value=0
  GPS Month : Outport
  GPS Day : Outport  Port=2
  GPS Year : Outport  Port=3
  GPS Hr : Outport  Port=4
  GPS Min : Outport  Port=5
  GPS Sec : Outport  Port=6
  GPS Frac Sec : Outport  Port=7
  GPS Lat (rad) : Outport  Port=8
  GPS Long (rad) : Outport  Port=9
  GPS H (m) : Outport  Port=10
  wires:
  NEU2NED/1 -> Flat Earth to LLA/1
  Zero level trust/1 -> Flat Earth to LLA/2
  XYZ (NEU)/1 -> NEU2NED/1
  Flat Earth to LLA/1 -> Angle Conversion/1
  Flat Earth to LLA/2 -> GPS H (m)/1
  Zero level trust1/1 -> MATLAB Fcn/1
  MATLAB Fcn/1 -> Demux/1
  Demux/2 -> GPS Month/1
  Demux/3 -> GPS Day/1
  Demux/1 -> GPS Year/1
  Demux/4 -> GPS Hr/1
  Demux/5 -> GPS Min/1
  Demux/6 -> Rounding Function/1
  Rounding Function/1 -> GPS Sec/1
  Zero level trust2/1 -> GPS Frac Sec/1
  Angle Conversion/1 -> Demux2/1
  Demux2/1 -> GPS Lat (rad)/1
  Demux2/2 -> GPS Long (rad)/1

== system PositionComplementary2/Plant Model/Plant/ISA Atmosphere & Winds ==
  "X, Y, Z" : Inport
  Correct Wind : Constant  Value=[0;0;0]
  Get Z : Selector  IndexOptions=Index vector (dialog)  Indices=[3]  OutputSizes=[(-2)]  InputPortWidth=3
  ISA Atmosphere Model1 : aerolibatmos2/ISA Atmosphere Model  SystemSampleTime=-1  custom=off  g=9.80665  gamma=1.4  R=287.0531  L=0.0065  h_trop=11000  h_strat=20000  rho0=1.225  P0=101325  T0=288.15
  Terminator : Terminator
  Terminator1 : Terminator
  Rho : Outport
  Wind : Outport  Port=2
  AirPressure (Pa) : Outport  Port=3
  wires:
  "X, Y, Z"/1 -> Get Z/1
  Get Z/1 -> ISA Atmosphere Model1/1
  ISA Atmosphere Model1/4 -> Rho/1
  ISA Atmosphere Model1/1 -> Terminator/1
  ISA Atmosphere Model1/2 -> Terminator1/1
  ISA Atmosphere Model1/3 -> AirPressure (Pa)/1
  Correct Wind/1 -> Wind/1

== system PositionComplementary2/Position  Complementary Filter/Subsystem/RB2LTP ==
  Euler : Inport
  11 : Fcn  Expr=cos(u[3])*cos(u[2])
  12 : Fcn  Expr=sin(u[3])*cos(u[2])
  13 : Fcn  Expr=-sin(u[2])
  21 : Fcn  Expr=cos(u[3])*sin(u[2])*sin(u[1])-sin(u[3])*cos(u[1])
  22 : Fcn  Expr=sin(u[3])*sin(u[2])*sin(u[1])+cos(u[3])*cos(u[1])
  23 : Fcn  Expr=cos(u[2])*sin(u[1])
  31 : Fcn  Expr=cos(u[3])*sin(u[2])*cos(u[1])+sin(u[3])*sin(u[1])
  32 : Fcn  Expr=sin(u[3])*sin(u[2])*cos(u[1])-cos(u[3])*sin(u[1])
  33 : Fcn  Expr=cos(u[2])*cos(u[1])
  Mux2 : Mux  Inputs=9
  Reshape : Reshape  OutputDimensionality=Customize  OutputDimensions=[3,3]
  Rot : Outport
  wires:
  Reshape/1 -> Rot/1
  Euler/1 -> 12/1, 13/1, 21/1, 22/1, 23/1, 31/1, 32/1, 33/1, 11/1
  Mux2/1 -> Reshape/1
  11/1 -> Mux2/1
  12/1 -> Mux2/2
  13/1 -> Mux2/3
  21/1 -> Mux2/4
  22/1 -> Mux2/5
  23/1 -> Mux2/6
  31/1 -> Mux2/7
  32/1 -> Mux2/8
  33/1 -> Mux2/9

== system PositionComplementary2/Signal Cond/Accel Convert/3vector LPF ==
  In1 : Inport  Orientation=left
  Demux : Demux  Orientation=left  Outputs=3
  Low Pass1 : Subsystem  Orientation=left  mask(DiscretizedZeroPole){Zeros=[], Poles=[-flpf], Gain=flpf, AbsTol=auto, SampleTime=SampleT, method=tustin, Wc=1}
      mask prompts: Zeros "Zeros (enter in s-main:)"; Poles "Poles (enter in s-domain:)"; Gain "Gain (enter in s-domain:)"; AbsTol "Absolute tolerance:"; SampleTime "Sample time:"; Wc "Critical Frequency (Hz):"
      mask help: Continuous mask uses c2d to transform parameters onto the Discrete Zero-Pole block inside.
      mask init:
      | st=SampleTime;
      | if length(st)>1
      |     st=SampleTime(1);
      | end
      | if(st>0)
      |     [zerosd,polesd,gaind] = sldiscutil('disczpk', {st,method,Wc,Zeros,Poles,Gain});
      | end	
      | s = get_param(gcb,'maskvalues');
      | zeross = s{1};
      | poless = s{2};
      | gainss = s{3};
      | %zerosc = eval(zeross);
      | %polesc = eval(poless);
      | %gainsc = eval(gainss);
      | sldiscutil('initzpkmask', st);
      | if(st==0)
      | set_param([gcb '/Zero Pole'], 'AbsoluteTolerance', AbsTol);
      | end
      mask StyleString: edit,edit,edit,edit,edit,popup(zoh|foh|tustin|prewarp|matched),edit
      mask CallbackString: |||||hidecrit|
      mask Display:
      | droots(zeross,poless,gainss)
      | text( 0.5, 1.0, method, 'verticalAlignment','top')
  Low Pass2 : Subsystem  Orientation=left  mask(DiscretizedZeroPole){Zeros=[], Poles=[-flpf], Gain=flpf, AbsTol=auto, SampleTime=SampleT, method=tustin, Wc=1}
      mask prompts: Zeros "Zeros (enter in s-main:)"; Poles "Poles (enter in s-domain:)"; Gain "Gain (enter in s-domain:)"; AbsTol "Absolute tolerance:"; SampleTime "Sample time:"; Wc "Critical Frequency (Hz):"
      mask help: Continuous mask uses c2d to transform parameters onto the Discrete Zero-Pole block inside.
      mask init: same as PositionComplementary2/Signal Cond/Accel Convert/3vector LPF/Low Pass1
      mask StyleString: edit,edit,edit,edit,edit,popup(zoh|foh|tustin|prewarp|matched),edit
      mask CallbackString: |||||hidecrit|
      mask Display:
      | droots(zeross,poless,gainss)
      | text( 0.5, 1.0, method, 'verticalAlignment','top')
  Low Pass3 : Subsystem  Orientation=left  mask(DiscretizedZeroPole){Zeros=[], Poles=[-flpf], Gain=flpf, AbsTol=auto, SampleTime=SampleT, method=tustin, Wc=1}
      mask prompts: Zeros "Zeros (enter in s-main:)"; Poles "Poles (enter in s-domain:)"; Gain "Gain (enter in s-domain:)"; AbsTol "Absolute tolerance:"; SampleTime "Sample time:"; Wc "Critical Frequency (Hz):"
      mask help: Continuous mask uses c2d to transform parameters onto the Discrete Zero-Pole block inside.
      mask init: same as PositionComplementary2/Signal Cond/Accel Convert/3vector LPF/Low Pass1
      mask StyleString: edit,edit,edit,edit,edit,popup(zoh|foh|tustin|prewarp|matched),edit
      mask CallbackString: |||||hidecrit|
      mask Display:
      | droots(zeross,poless,gainss)
      | text( 0.5, 1.0, method, 'verticalAlignment','top')
  Mux : Mux  Orientation=left  Inputs=3
  Out1 : Outport  Orientation=left
  wires:
  Demux/1 -> Low Pass1/1(In1)
  Demux/2 -> Low Pass2/1(In1)
  Demux/3 -> Low Pass3/1(In1)
  Low Pass1/1(Out1) -> Mux/1
  Low Pass2/1(Out1) -> Mux/2
  Low Pass3/1(Out1) -> Mux/3
  In1/1 -> Demux/1
  Mux/1 -> Out1/1

== system PositionComplementary2/Signal Cond/Gyro Convert/3vector LPF ==
  In1 : Inport  Orientation=left
  Demux : Demux  Orientation=left  Outputs=3
  Low Pass1 : Subsystem  Orientation=left  mask(DiscretizedZeroPole){Zeros=[], Poles=[-flpf], Gain=flpf, AbsTol=auto, SampleTime=SampleT, method=tustin, Wc=1}
      mask prompts: Zeros "Zeros (enter in s-main:)"; Poles "Poles (enter in s-domain:)"; Gain "Gain (enter in s-domain:)"; AbsTol "Absolute tolerance:"; SampleTime "Sample time:"; Wc "Critical Frequency (Hz):"
      mask help: Continuous mask uses c2d to transform parameters onto the Discrete Zero-Pole block inside.
      mask init: same as PositionComplementary2/Signal Cond/Accel Convert/3vector LPF/Low Pass1
      mask StyleString: edit,edit,edit,edit,edit,popup(zoh|foh|tustin|prewarp|matched),edit
      mask CallbackString: |||||hidecrit|
      mask Display:
      | droots(zeross,poless,gainss)
      | text( 0.5, 1.0, method, 'verticalAlignment','top')
  Low Pass2 : Subsystem  Orientation=left  mask(DiscretizedZeroPole){Zeros=[], Poles=[-flpf], Gain=flpf, AbsTol=auto, SampleTime=SampleT, method=tustin, Wc=1}
      mask prompts: Zeros "Zeros (enter in s-main:)"; Poles "Poles (enter in s-domain:)"; Gain "Gain (enter in s-domain:)"; AbsTol "Absolute tolerance:"; SampleTime "Sample time:"; Wc "Critical Frequency (Hz):"
      mask help: Continuous mask uses c2d to transform parameters onto the Discrete Zero-Pole block inside.
      mask init: same as PositionComplementary2/Signal Cond/Accel Convert/3vector LPF/Low Pass1
      mask StyleString: edit,edit,edit,edit,edit,popup(zoh|foh|tustin|prewarp|matched),edit
      mask CallbackString: |||||hidecrit|
      mask Display:
      | droots(zeross,poless,gainss)
      | text( 0.5, 1.0, method, 'verticalAlignment','top')
  Low Pass3 : Subsystem  Orientation=left  mask(DiscretizedZeroPole){Zeros=[], Poles=[-flpf], Gain=flpf, AbsTol=auto, SampleTime=SampleT, method=tustin, Wc=1}
      mask prompts: Zeros "Zeros (enter in s-main:)"; Poles "Poles (enter in s-domain:)"; Gain "Gain (enter in s-domain:)"; AbsTol "Absolute tolerance:"; SampleTime "Sample time:"; Wc "Critical Frequency (Hz):"
      mask help: Continuous mask uses c2d to transform parameters onto the Discrete Zero-Pole block inside.
      mask init: same as PositionComplementary2/Signal Cond/Accel Convert/3vector LPF/Low Pass1
      mask StyleString: edit,edit,edit,edit,edit,popup(zoh|foh|tustin|prewarp|matched),edit
      mask CallbackString: |||||hidecrit|
      mask Display:
      | droots(zeross,poless,gainss)
      | text( 0.5, 1.0, method, 'verticalAlignment','top')
  Mux : Mux  Orientation=left  Inputs=3
  Out1 : Outport  Orientation=left
  wires:
  Demux/1 -> Low Pass1/1(In1)
  Demux/2 -> Low Pass2/1(In1)
  Demux/3 -> Low Pass3/1(In1)
  Low Pass1/1(Out1) -> Mux/1
  Low Pass2/1(Out1) -> Mux/2
  Low Pass3/1(Out1) -> Mux/3
  In1/1 -> Demux/1
  Mux/1 -> Out1/1
